simulink model "control"  (R2022b)
settings: Solver=VariableStepAuto  StartTime=0.0  StopTime=10.0  RelTol=1e-3
values from neighbouring files (symbols this model uses):
  q0 = [-0.9273 -1.287 0.7 2.2143]    [generated_traj.mat]
  Tc = 0.001    [generated_traj.mat]
undefined symbols (not defined in the file or in its folder): DiscIntNeverNeededParam
settings Model: Creator=giuseppeloianno  LastModifiedBy=CHINMAY PRASHANTH

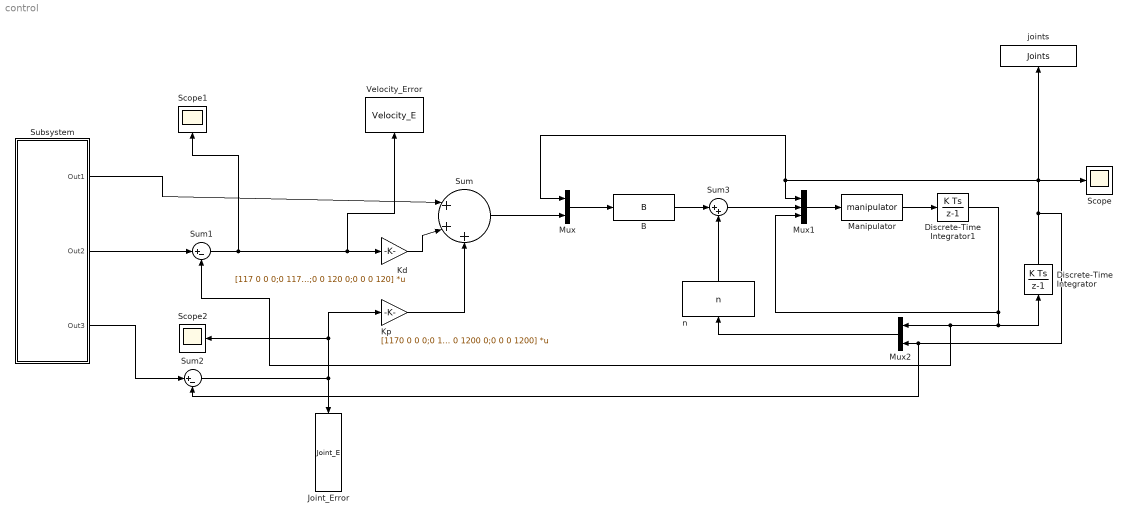
== system control ==
  B : MATLABFcn  MATLABFcn=B  OutputDimensions=4
  Discrete-Time Integrator : DiscreteIntegrator  InitialCondition=q0  SampleTime=Tc  LimitOutput=on  UpperSaturationLimit=[inf;inf;inf;inf]  LowerSaturationLimit=[-inf;-inf;-inf;-inf]  ICPrevOutput=DiscIntNeverNeededParam  ICPrevScaledInput=DiscIntNeverNeededParam
  Discrete-Time Integrator1 : DiscreteIntegrator  InitialCondition=q0  SampleTime=0.001  ICPrevOutput=DiscIntNeverNeededParam  ICPrevScaledInput=DiscIntNeverNeededParam
  Joint_Error : ToWorkspace  VariableName=Joint_E  SampleTime=-1
  Kd : Gain  Gain=[117 0 0 0;0 117 0 0;0 0 120 0;0 0 0 120]  Multiplication=Matrix(K*u)
  Kp : Gain  Gain=[1170 0 0 0;0 1170 0 0;0 0 1200 0;0 0 0 1200]  Multiplication=Matrix(K*u)
  Manipulator : MATLABFcn  MATLABFcn=manipulator  OutputDimensions=4
  Mux : Mux  Inputs=2
  Mux1 : Mux  Inputs=3
  Mux2 : Mux  Inputs=2
  Scope : Scope
  Scope1 : Scope
  Scope2 : Scope
  Subsystem : Subsystem
  Sum : Sum  Inputs=|+++
  Sum1 : Sum  Inputs=|+-
  Sum2 : Sum  Inputs=|+-
  Sum3 : Sum  Inputs=|++
  Velocity_Error : ToWorkspace  VariableName=Velocity_E  SampleTime=-1
  joints : ToWorkspace  VariableName=Joints  SampleTime=-1
  n : MATLABFcn  MATLABFcn=n  OutputDimensions=4
  wires:
  Mux1/1 -> Manipulator/1
  Mux/1 -> B/1
  Mux2/1 -> n/1
  Manipulator/1 -> Discrete-Time Integrator1/1
  Sum/1 -> Mux/2
  Sum2/1 -> Kp/1, Scope2/1, Joint_Error/1
  Kp/1 -> Sum/3
  n/1 -> Sum3/2
  Discrete-Time Integrator/1 -> Mux/1, Mux1/1, joints/1, Scope/1, Mux2/2, Sum2/2
  Discrete-Time Integrator1/1 -> Mux1/3, Mux2/1, Sum1/2, Discrete-Time Integrator/1
  Sum3/1 -> Mux1/2
  Kd/1 -> Sum/2
  B/1 -> Sum3/1
  Subsystem/1(Out1) -> Sum/1
  Sum1/1 -> Velocity_Error/1, Kd/1, Scope1/1
  Subsystem/2(Out2) -> Sum1/1
  Subsystem/3(Out3) -> Sum2/1

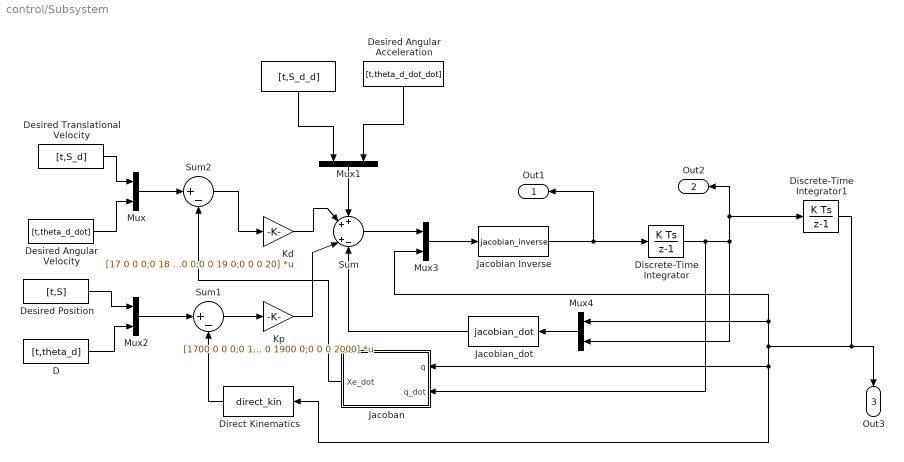
== system control/Subsystem ==
  " " : FromWorkspace  VariableName=[t,S_d_d]  SampleTime=0.001
  D : FromWorkspace  VariableName=[t,theta_d]  SampleTime=0.001
  Desired Angular Acceleration : FromWorkspace  VariableName=[t,theta_d_dot_dot]  SampleTime=0.001
  Desired Angular Velocity : FromWorkspace  VariableName=[t,theta_d_dot]  SampleTime=0.001
  Desired Position : FromWorkspace  VariableName=[t,S]  SampleTime=0.001
  Desired Translational Velocity : FromWorkspace  VariableName=[t,S_d]  SampleTime=0.001
  Direct Kinematics : MATLABFcn  MATLABFcn=direct_kin  OutputDimensions=4
  Discrete-Time Integrator : DiscreteIntegrator  InitialCondition=q0  SampleTime=Tc  ICPrevOutput=DiscIntNeverNeededParam  ICPrevScaledInput=DiscIntNeverNeededParam
  Discrete-Time Integrator1 : DiscreteIntegrator  InitialCondition=q0  SampleTime=Tc  ICPrevOutput=DiscIntNeverNeededParam  ICPrevScaledInput=DiscIntNeverNeededParam
  "Jacoban " : MATLAB Function  TreatAsAtomicUnit=on
  Jacobian Inverse : MATLABFcn  MATLABFcn=jacobian_inverse  OutputDimensions=4
  Jacobian_dot : MATLABFcn  MATLABFcn=jacobian_dot  OutputDimensions=4
  Kd : Gain  Gain=[17 0 0 0;0 18 0 0;0 0 19 0;0 0 0 20]  Multiplication=Matrix(K*u)
  Kp : Gain  Gain=[1700 0 0 0;0 1800 0 0;0 0 1900 0;0 0 0 2000]  Multiplication=Matrix(K*u)
  Mux{,1..4} (5 alike) : Mux  Inputs=2
  Sum : Sum  Inputs=++|+-
  Sum1 : Sum  Inputs=|+-
  Sum2 : Sum  Inputs=|+-
  Out1 : Outport
  Out2 : Outport  Port=2
  Out3 : Outport  Port=3
  wires:
  Direct Kinematics/1 -> Sum1/2
  Mux1/1 -> Sum/1
  Discrete-Time Integrator1/1 -> Direct Kinematics/1, "Jacoban "/1(q), Mux3/2, Mux4/1, Out3/1
  Jacobian Inverse/1 -> Discrete-Time Integrator/1, Out1/1
  " "/1 -> Mux1/1
  "Jacoban "/1(Xe_dot) -> Sum2/2
  Kd/1 -> Sum/2
  Desired Translational Velocity/1 -> Mux/1
  Mux4/1 -> Jacobian_dot/1
  Jacobian_dot/1 -> Sum/4
  Discrete-Time Integrator/1 -> Mux4/2, Discrete-Time Integrator1/1, Out2/1, "Jacoban "/2(q_dot)
  Mux/1 -> Sum2/1
  D/1 -> Mux2/2
  Mux3/1 -> Jacobian Inverse/1
  Mux2/1 -> Sum1/1
  Kp/1 -> Sum/3
  Desired Angular Velocity/1 -> Mux/2
  Sum/1 -> Mux3/1
  Sum2/1 -> Kd/1
  Sum1/1 -> Kp/1
  Desired Position/1 -> Mux2/1
  Desired Angular Acceleration/1 -> Mux1/2

== matlab function control/Subsystem/Jacoban  ==
  data: q input; Xe_dot output; q_dot input
function Xe_dot= fcn(q,q_dot)


    theta1=q(1);
    theta2=q(2);
    
    a1=0.5;
    
    a2=0.5;
    
    Jacobian=[- a2*sin(theta1 + theta2) - a1*sin(theta1), -a2*sin(theta1 + theta2), 0, 0; 
        a2*cos(theta1 + theta2) + a1*cos(theta1), a2*cos(theta1 + theta2), 0,0; 
        0, 0, -1, 0;
        1, 1, 0, 1];
    
    Xe_dot=Jacobian*q_dot;

end
